simulink model "convert_ex"  (R2020a)
settings: Solver=VariableStepAuto  StartTime=0.0  StopTime=10.0  RelTol=1e-3
settings Model: Creator=lenovo  LastModifiedBy=DELL
settings DataIOCC: ReturnWorkspaceOutputs=off
settings DebuggingCC: ArithmeticOperatorsInVariantConditions=warning
settings SFSimCC: SimUseLocalCustomCode=off  CustomCodeUndefinedFunction=UseInterfaceOnly
settings RTWCC: RTWUseLocalCustomCode=off

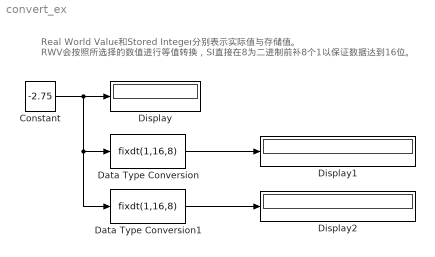
== system convert_ex ==
  note: Real World Value和Stored Integer分别表示实际值与存储值。
      | RWV会按照所选择的数值进行等值转换，SI直接在8为二进制前补8个1以保证数据达到16位。
  Constant : Constant  Value=-2.75  OutDataTypeStr=fixdt(1,8,3)
  Data Type Conversion : DataTypeConversion  OutDataTypeStr=fixdt(1,16,8)
  Data Type Conversion1 : DataTypeConversion  OutDataTypeStr=fixdt(1,16,8)  ConvertRealWorld=Stored Integer (SI)
  Display : Display
      settings: Format=binary (Stored Integer)
  Display1 : Display
      settings: Format=binary (Stored Integer)
  Display2 : Display
      settings: Format=binary (Stored Integer)
  wires:
  Constant/1 -> Data Type Conversion1/1, Data Type Conversion/1, Display/1
  Data Type Conversion/1 -> Display1/1
  Data Type Conversion1/1 -> Display2/1
